simulink model "Zoh"  (R2023a)
settings: Solver=VariableStepAuto  StartTime=0.0  StopTime=10.0  RelTol=1e-3
settings Model: Creator=Georgiy  LastModifiedBy=Georgiy

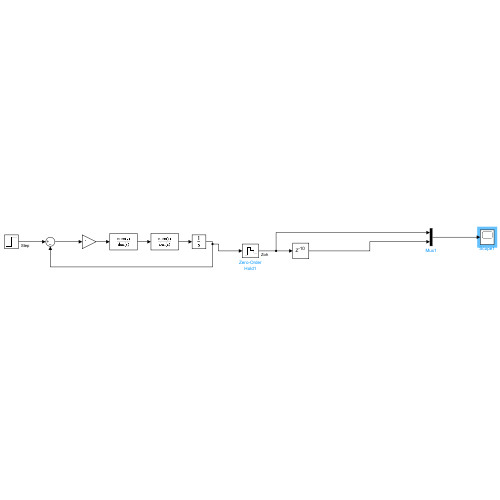
[thumbnail: Simulink's stored preview of the top-level diagram]
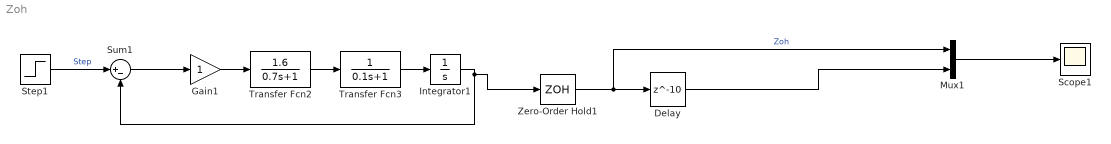
== system Zoh ==
  Delay : Delay  DelayLength=10  InitialCondition=0  SampleTime=0.2
  Gain1 : Gain
  Integrator1 : Integrator
  Mux1 : Mux  Inputs=2
  Scope1 : Scope
  Step1 : Step  SampleTime=0
  Sum1 : Sum  Inputs=|+-
  Transfer Fcn2 : TransferFcn  Numerator=[1.6]  Denominator=[0.7 1]
  Transfer Fcn3 : TransferFcn  Denominator=[0.1 1]
  Zero-Order Hold1 : ZeroOrderHold  SampleTime=-1
  wires:
  Transfer Fcn3/1 -> Integrator1/1
  Gain1/1 -> Transfer Fcn2/1
  Step1/1 -> Sum1/1  "Step"
  Zero-Order Hold1/1 -> Delay/1, Mux1/1  "Zoh"
  Sum1/1 -> Gain1/1
  Mux1/1 -> Scope1/1
  Integrator1/1 -> Sum1/2, Zero-Order Hold1/1
  Transfer Fcn2/1 -> Transfer Fcn3/1
  Delay/1 -> Mux1/2
